simulink model "motion_3D_1_2_w12_5"  (R2025b)
settings: Solver=FixedStepAuto  StartTime=0.0  StopTime=3.5  FixedStep=Ts  RelTol=1e-3
values from neighbouring files (symbols this model uses):
  Ts = 1/1600    (= 0.000625)    [path_control.m]    (also in run_case1.m; run_case1_Cdx.m; run_simulation.m = params.common.Ts; verify_eq12_spectral_PP.m)
libraries: simulink x1, slpidlib x1
settings Model: Creator=user  LastModifiedBy=PME406_01
settings SolverCC: AlgebraicLoopSolver=LineSearch
settings DataIOCC: SaveFormat=Array  ReturnWorkspaceOutputs=off
settings DebuggingCC: UnconnectedInputMsg=warning  UnconnectedOutputMsg=warning  UnconnectedLineMsg=warning  ArithmeticOperatorsInVariantConditions=warning
settings ModelReferenceCC: EnableRefExpFcnMdlSchedulingChecks=on
settings SFSimCC: SimUseLocalCustomCode=off  CustomCodeUndefinedFunction=UseInterfaceOnly
settings RTWCC: RTWUseLocalCustomCode=off  GPUComputeCapability=3.5
settings CodeAppCC: StateflowObjectComments=on

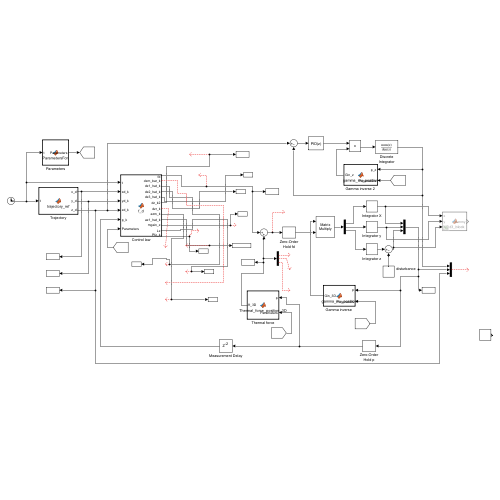
[thumbnail: Simulink's stored preview of the top-level diagram]
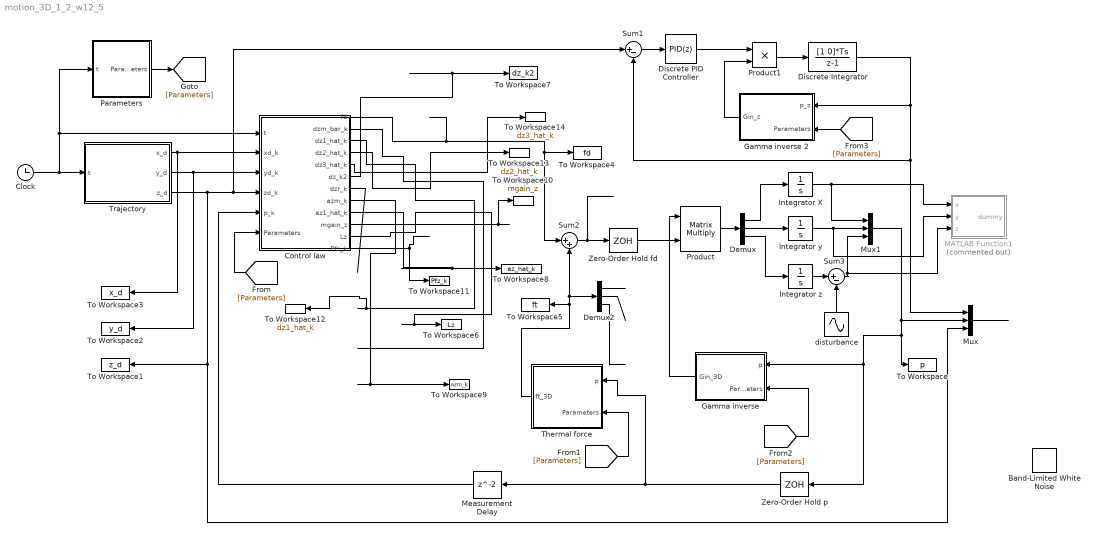
== system motion_3D_1_2_w12_5 ==
  Band-Limited White Noise : simulink/Sources/Band-Limited White Noise  Cov=[0.1]  Ts=0.1  seed=[23341]
  Clock : Clock
  Control law : MATLAB Function  TreatAsAtomicUnit=on
  Demux : Demux  Outputs=3
  Demux2 : Demux  Outputs=3
  Discrete Integrator : DiscreteTransferFcn  Numerator=[1 0]*Ts  Denominator=[1 -1]  SampleTime=Ts
  Discrete PID Controller : slpidlib/PID Controller  Controller=PID  Form=Parallel  TimeDomain=Discrete-time  UseExternalTs=off  SampleTime=Ts  IntegratorMethod=Forward Euler  FilterMethod=Forward Euler  ControllerParametersSource=internal  P=1  I=1  UseKiTs=off  D=0  UseExternalDerivativeSource=off  N=31.4504174128775  UseFilter=on  TunerSelectOption=Transfer Function Based (PID Tuner App)  InitialConditionSource=internal  InitialConditionForIntegrator=0  InitialConditionForFilter=0  DifferentiatorICPrevScaledInput=0  ExternalReset=none  TrackingMode=off  Kt=1  LimitOutput=off  SatLimitsSource=internal  UpperSaturationLimit=inf  LowerSaturationLimit=-inf  LinearizeAsGain=off  AntiWindupMode=none  Kb=1  LimitIntegrator=off  UpperIntegratorSaturationLimit=inf  LowerIntegratorSaturationLimit=-inf  POutMin=[]  POutMax=[]  IOutMin=[]  IOutMax=[]  DOutMin=[]  DOutMax=[]  NOutMin=[]  NOutMax=[]  SumOutMin=[]  SumOutMax=[]  SaturationOutMin=[]  SaturationOutMax=[]  PParamMin=[]  PParamMax=[]  IParamMin=[]  IParamMax=[]  DParamMin=[]  DParamMax=[]  NParamMin=[]  NParamMax=[]  KbParamMin=[]  KbParamMax=[]  KtParamMin=[]  KtParamMax=[]  KbOutMin=[]  KbOutMax=[]  KtOutMin=[]  KtOutMax=[]  IntegratorOutMin=[]  IntegratorOutMax=[]  FilterOutMin=[]  FilterOutMax=[]  SumI1OutMin=[]  SumI1OutMax=[]  SumI2OutMin=[]  SumI2OutMax=[]  SumI3OutMin=[]  SumI3OutMax=[]  SumI4OutMin=[]  SumI4OutMax=[]  SumDOutMin=[]  SumDOutMax=[]  DifferentiatorOutMin=[]  DifferentiatorOutMax=[]  FilterDiffOutCoefMin=[]  FilterDiffOutCoefMax=[]  ReciprocalOutMin=[]  ReciprocalOutMax=[]  SumDenOutMin=[]  SumDenOutMax=[]  SumNumOutMin=[]  SumNumOutMax=[]  DivideOutMin=[]  DivideOutMax=[]  UdiffTsProdOutMin=[]  UdiffTsProdOutMax=[]  NTsProdOutMin=[]  NTsProdOutMax=[]  UintegralTsProdOutMin=[]  UintegralTsProdOutMax=[]  UngainTsProdOutMin=[]  UngainTsProdOutMax=[]  ClampingZeroOutDataTypeStr=Inherit: Inherit via back propagation  ClampingZeroOutMin=[]  ClampingZeroOutMax=[]  FilterDenConstantOutDataTypeStr=Inherit: Inherit via back propagation  FilterDenConstantOutMin=[]  FilterDenConstantOutMax=[]  PCopyOutDataTypeStr=Inherit: Inherit via back propagation  PCopyOutMin=[]  PCopyOutMax=[]  NCopyOutDataTypeStr=Inherit: Inherit via back propagation  NCopyOutMin=[]  NCopyOutMax=[]  IntegratorContinuousStateAttributes=''  IntegratorStateMustResolveToSignalObject=off  IntegratorRTWStateStorageClass=Auto  FilterContinuousStateAttributes=''  FilterStateMustResolveToSignalObject=off  FilterRTWStateStorageClass=Auto  ParallelPVariant=InternalParameters  IdealPVariant=Disabled  IVariant=InternalParameters  DVariant=InternalParameters  IntegratorVariant=Discrete  SatVariant=Disabled  AWVariant=Passthrough  PCopyVariant=Disabled  TRVariant=Disabled  FdbkBlocksVariant=Forward  IdealPFdbkVariant=Disabled  SatFdbkVariant=Disabled  DerivativeFilterVariant=ForwardEulerFilter  NVariant=InternalParameters  NCopyVariant=Disabled  FilterICVariant=InternalICsFilter  IntegratorICVariant=InternalICs  ExternalResetVariant=Disabled  TRSumVariant=Passthrough  SumFdbkVariant=Disabled  SumVariant=Sum_PID  TsampFilterVariant=InternalTs  TsampNgainVariant=Passthrough  TsampIntegralVariant=Disabled_SignalSpec  ExternalSaturationOutDataTypeStr=Inherit: Same as second input  DerivativeSourceVariant=ErrorSignal  PreIntVariant=InternalPreInt
  "Gamma inverse " : MATLAB Function  TreatAsAtomicUnit=on
  "Gamma inverse 2 " : MATLAB Function  TreatAsAtomicUnit=on
  Integrator X : Integrator
  Integrator y : Integrator
  Integrator z : Integrator
  MATLAB Function1 : MATLAB Function  Commented=on  TreatAsAtomicUnit=on
  Measurement Delay : Delay  SampleTime=Ts
  Mux : Mux  Inputs=3
  Mux1 : Mux  Inputs=3
  Parameters : MATLAB Function  TreatAsAtomicUnit=on
  Product : Product  Multiplication=Matrix(*)
  Product1 : Product
  Sum1 : Sum  Inputs=|+-
  Sum2 : Sum  Inputs=|++
  Sum3 : Sum  Inputs=|+-
  "Thermal force " : MATLAB Function  TreatAsAtomicUnit=on
  To Workspace : ToWorkspace  VariableName=p  SampleTime=Ts
  To Workspace1 : ToWorkspace  VariableName=z_d  SampleTime=Ts
  To Workspace10 : ToWorkspace  VariableName=mgain_z  SampleTime=Ts
  To Workspace11 : ToWorkspace  VariableName=Pfz_k  SampleTime=Ts
  To Workspace12 : ToWorkspace  VariableName=dz1_hat_k  SampleTime=Ts
  To Workspace13 : ToWorkspace  VariableName=dz2_hat_k  SampleTime=Ts
  To Workspace14 : ToWorkspace  VariableName=dz3_hat_k  SampleTime=Ts
  To Workspace2 : ToWorkspace  VariableName=y_d  SampleTime=Ts
  To Workspace3 : ToWorkspace  VariableName=x_d  SampleTime=Ts
  To Workspace4 : ToWorkspace  VariableName=fd  SampleTime=Ts
  To Workspace5 : ToWorkspace  VariableName=ft  SampleTime=Ts
  To Workspace6 : ToWorkspace  VariableName=Lz  SampleTime=Ts
  To Workspace7 : ToWorkspace  VariableName=dz_k2  SampleTime=Ts
  To Workspace8 : ToWorkspace  VariableName=az_hat_k  SampleTime=Ts
  To Workspace9 : ToWorkspace  VariableName=azm_k  SampleTime=Ts
  Trajectory : MATLAB Function  TreatAsAtomicUnit=on
  Zero-Order Hold fd : ZeroOrderHold  SampleTime=Ts
  Zero-Order Hold p : ZeroOrderHold  SampleTime=Ts
  "disturbance " : Sin  Amplitude=0*10^-6  Frequency=2*pi*10  Phase=pi/2  SampleTime=Ts
  wires:
  Mux/1 -> ?
  Product1/1 -> Discrete Integrator/1
  Integrator z/1 -> Sum3/1
  Sum3/1 -> MATLAB Function1/3(z), Mux1/3
  Sum1/1 -> Discrete PID Controller/1
  Discrete PID Controller/1 -> Product1/1
  Measurement Delay/1 -> Control law/5(p_k)
  Integrator X/1 -> Mux1/1, MATLAB Function1/1(x)
  Mux1/1 -> Zero-Order Hold p/1, "Gamma inverse "/1(p), To Workspace/1, Mux/2
  Control law/1(fd) -> Sum2/1, To Workspace4/1
  "disturbance "/1 -> Sum3/2
  Integrator y/1 -> MATLAB Function1/2(y), Mux1/2
  Clock/1 -> Parameters/1(t), Control law/1(t), Trajectory/1(t)
  Trajectory/2(y_d) -> To Workspace2/1, Control law/3(yd_k)
  Trajectory/3(z_d) -> Mux/3, To Workspace1/1, Control law/4(zd_k), Sum1/1
  Discrete Integrator/1 -> Mux/1, Sum1/2, "Gamma inverse 2 "/1(p_z)
  Product/1 -> Demux/1
  Trajectory/1(x_d) -> To Workspace3/1, Control law/2(xd_k)
  Demux/1 -> Integrator X/1
  Demux/2 -> Integrator y/1
  Demux/3 -> Integrator z/1
  Zero-Order Hold fd/1 -> Product/2
  Zero-Order Hold p/1 -> "Thermal force "/1(p), Measurement Delay/1
  Sum2/1 -> Zero-Order Hold fd/1
  Demux2/1 -> ?
  Demux2/2 -> ?
  Demux2/3 -> ?
  Control law/6(dz_k2) -> To Workspace7/1
  Control law/2(dzm_bar_k) -> ?
  Control law/7(dzr_k) -> ?
  Control law/3(dz1_hat_k) -> To Workspace12/1
  Control law/8(azm_k) -> To Workspace9/1
  Control law/9(az1_hat_k) -> To Workspace8/1
  Control law/11(Lz) -> To Workspace6/1
  Control law/10(mgain_z) -> To Workspace10/1
  Control law/12(Pfz_k) -> To Workspace11/1
  Control law/4(dz2_hat_k) -> To Workspace13/1
  Control law/5(dz3_hat_k) -> To Workspace14/1
  "Thermal force "/1(ft_3D) -> To Workspace5/1, Demux2/1, Sum2/2
  Parameters/1(Parameters) -> [Parameters]
  [Parameters] -> Control law/6(Parameters)
  [Parameters] -> "Thermal force "/2(Parameters)
  "Gamma inverse "/1(Gin_3D) -> Product/1
  [Parameters] -> "Gamma inverse "/2(Parameters)
  "Gamma inverse 2 "/1(Gin_z) -> Product1/2
  [Parameters] -> "Gamma inverse 2 "/2(Parameters)

== matlab function motion_3D_1_2_w12_5/MATLAB Function1 ==
  data: x input; dummy output; y input; z input
function dummy = plot3_block(x, y, z)
% 用於模擬時即時顯示 3D 點 / 轨跡

% 告訴 codegen：這些函式只在模擬時呼叫
%coder.extrinsic('plot3','figure','hold','grid','xlabel','ylabel','zlabel',...
%                'get','set','drawnow');
coder.extrinsic('plot3','figure','hold','grid','xlabel','ylabel','zlabel',...
                'get','set','drawnow','axis','xlim','ylim','zlim','view','rotate3d');
persistent h
persistent isInit

if isempty(isInit)
    figure; hold on; grid on;
    xlabel('x'); ylabel('y'); zlabel('z');
    axis equal;                   % 三個方向比例一樣
    xlim([-1 1]*4*10^1);                 % 自己設定範圍（依你的資料）
    ylim([-1 1]*4*10^1);
    zlim([-1 1]*4*10^1);
    view(3);                      % 確認使用 3D 視角
    rotate3d on;
    
    % 先畫第一個點，取得圖形 handle
    h = plot3(x, y, z, '.-');
    isInit = true;
else
    % 讀取舊資料，把新的點接到後面
    X = get(h, 'XData');  Y = get(h, 'YData');  Z = get(h, 'ZData');
    X = [X x];  Y = [Y y];  Z = [Z z];
    set(h, 'XData', X, 'YData', Y, 'ZData', Z);
end

drawnow;          % 更新圖形
dummy = 0;        % 給一個不重要的輸出
end

== matlab function motion_3D_1_2_w12_5/Control law ==
  settings: updateMethod=DISCRETE  sampleTime=Ts
  data: t input; xd_k input; yd_k input; zd_k input; fd output size=[3 1]; p_k input size=[3 1]; dzm_bar_k output; dz1_hat_k output; dz2_hat_k output; dz3_hat_k output; dz_k2 output; dzr_k output; azm_k output; az1_hat_k output; mgain_z output; Lz output; Pfz_k output; Parameters input
function [fd, dzm_bar_k, dz1_hat_k, dz2_hat_k, dz3_hat_k, dz_k2 , dzr_k , azm_k , az1_hat_k , mgain_z , Lz , Pfz_k] = f_d(t, xd_k,yd_k,zd_k, p_k, Parameters)

% xd_k : x_d[k]
% xd_k1  : x_d[k-1]
% x_k   : x[k]
% fd    : f_d[k]
% ====================================================================
% PERSISTENT STATE VARIABLES
% ====================================================================
persistent xd_k1                 % x_d[k-1],         - Input history
persistent xd_k2
persistent yd_k1
persistent yd_k2
persistent zd_k1
persistent zd_k2
persistent px_k
persistent py_k
persistent pz_k
persistent fd_X
persistent fd_Y
persistent fd_Z

persistent        dx1_hat_k1
persistent        dx2_hat_k1 
persistent        dx3_hat_k1 
persistent        dz1_hat_k1
persistent        dz2_hat_k1 
persistent        dz3_hat_k1 
persistent        xD_hat_k1 
persistent        dxD_hat_k1
persistent        zD1_hat_k1 
persistent        zD2_hat_k1
persistent        ax_hat_k1 
persistent        ax_hat_k2
persistent        az1_hat_k1 
persistent        az1_hat_k2
persistent        dax_hat_k1 
persistent        az2_hat_k1 
persistent        Pfx_k1
persistent        Pfz_k1
persistent        fd_X_k1 
persistent        fd_X_k2
persistent        fd_Z_k1 
persistent        fd_Z_k2

persistent      dxm_bar_k1
persistent      dxr_bar_k1
persistent     dxr2_bar_k1
persistent      dzm_bar_k1
persistent      dzr_bar_k1
persistent     dzr2_bar_k1

persistent      px_k1
persistent      pz_k1
persistent      PPx_k1
persistent      PPz_k1
%persistent      dx_k1
%persistent      dx_k2
persistent      dx_k3
%persistent      dy_k1
%persistent      dy_k2
persistent      dy_k3
%persistent      dz_k1
%persistent      dz_k2
persistent      dz_k3
persistent      px_bar_k1
persistent      pz_bar_k1
persistent      dxrr_bar_k1
persistent      dzrr_bar_k1
persistent      dxm_k1
persistent      dzm_k1
persistent      azm_k1
% ====================================================================
% INITIALIZATION
% ====================================================================
    if isempty(xd_k1)
        xd_k1 = 0;     % 初始化（第一次執行時）
        xd_k2 = 0;
        yd_k1 = 0;
        yd_k2 = 0;
%        yd_k1 = 6.5;   %um  *10^-6;
        zd_k1 = 0;
        zd_k2 = 0;
        px_k = 0;
        py_k = 0;
        pz_k = 0;
        fd_X = 0;
        fd_Y = 0;
        fd_Z = 0;
        
         xD_hat_k1 = 0;
         
        dx1_hat_k1 = 0; 
        dx2_hat_k1 = 0;
        dx3_hat_k1 = 0;
        dz1_hat_k1 = 0; 
        dz2_hat_k1 = 0;
        dz3_hat_k1 = 0;
        
        xD_hat_k1 = 0;
        dxD_hat_k1 = 0;
        zD1_hat_k1 = 0;
        zD2_hat_k1 = 0;
        
        ax_hat_k1 = 0.012;   %( um/(pN sec))   %ax_normal = 0.0147*10^6; % ( m/(N sec))
        ax_hat_k2 = 0;
        az1_hat_k1 = 0.012/(1+Parameters.beta); % beta=0.5 %( um/(pN sec))        %az_normal = 0.0147*10^6; % ( m/(N sec))
        az_hat_k2 = 0;
        
        dax_hat_k1 = 0;
        az2_hat_k1 = 0;
        
        Pfx_k1 = (0.0147)*4*(1.3806503*10^-23)*(273.15 + 37)*diag([1 1 1 1 1 1 1])*1/4*10^-2;
        
        dz_variance = (2.3*10^-3)^2;    %(um)^2
        Pfz_11 = dz_variance; Pfz_22 = dz_variance;Pfz_33 = dz_variance;
        Pfz_44 = dz_variance;Pfz_55 = dz_variance;
        az_variance = (10^-1*az1_hat_k1)^2;
        Pfz_66 = az_variance; Pfz_77 = az_variance;
       % Pfz_k1 = diag([Pfz_11 Pfz_22 Pfz_33 Pfz_44 Pfz_55 Pfz_66 Pfz_77]);
        
       % simulation by experienced data
        Pfz_11 = Parameters.Pfz_11;
        Pfz_22 = Parameters.Pfz_22;
        Pfz_33 = Parameters.Pfz_33;
        Pfz_44 = Parameters.Pfz_44;
        Pfz_55 = Parameters.Pfz_55;
        Pfz_66 = Parameters.Pfz_66;
        Pfz_77 = Parameters.Pfz_77;
        Pfz_k1 = diag([Pfz_11 Pfz_22 Pfz_33 Pfz_44 Pfz_55 Pfz_66 Pfz_77]);
        
        dxm_bar_k1 = 0;
        dzm_bar_k1 = 0;
        dxr_bar_k1 = 0;
        dzr_bar_k1 = 0;
        dxrr_bar_k1 = 0;
        dzrr_bar_k1 = 0;
        
        dxr2_bar_k1 = 0.9*10^-15;
        
        dzr2_bar_k1 = (0.012*10^6)/Parameters.Am_scaling*4*Parameters.kb*Parameters.T*(2+1/(1-Parameters.lamdaC^2))*(10^6)^2; % (um)^2  ;  azm_n/azm_meas_factor* 4*kb*T * ( 2 + 1/(1 - lamdaC^2) );
        
        fd_X_k1 = 0;    %1*10^-12*10^6;
        fd_X_k2 = 0;
        fd_Z_k1 = 0;    %1*10^-12*10^6;
        fd_Z_k2 = 0;        
        
        px_k1 = 0;
        pz_k1 = 0;
        PPx_k1 = 4*(1.3806503*10^-23)*(273.15 + 37)*0.0147*10^38;        % 4*T*kB*t/g*10^38; da-min 
        PPz_k1 = 4*(1.3806503*10^-23)*(273.15 + 37)*0.0147*10^38;        % 4*T*kB*t/g*10^38;  da-min
%       dx_k1 = 0;     
%       dx_k2 = 0;
        dx_k3 = 0;
 %       dy_k1 = 0;     
 %       dy_k2 = 0;
        dy_k3 = 0;
 %       dz_k1 = 0;     
 %       dz_k2 = 0;
        dz_k3 = 0;        
        px_bar_k1 = 0;
        pz_bar_k1 = 0;
        dxm_k1 =  0;
        dzm_k1 =  0;
        
       azm_k1 = 0.012/Parameters.Am_scaling;  % ( um/(pN sec))   ;az_normal = 0.0147*10^6; %azm_meas_factor=2.5
    end
    
        Ts = Parameters.Ts;
        lamdaC = Parameters.lamdaC;
        gammaN = Parameters.gammaN;

        %parameters
        kb = Parameters.kb;
        T = Parameters.T;
        ax_normal = Parameters.ax_normal;
        az_normal = Parameters.az_normal;

        px_k = p_k(1);
        py_k = p_k(2);
        pz_k = p_k(3);

    % 1) Two angles and one distance defined the orientation and position of the inclined plane
    %theta = pi/2;
    %phi = 0;
    %pz = -15 *10^-6;
    theta = Parameters.theta;
    phi = Parameters.phi;
    pz = Parameters.pz;  

    % 2_1) Plane normal
    w_hat = [cos(theta)*sin(phi);
             sin(theta)*sin(phi);
             cos(phi)];
    % 2_2) Plane x-y unit vector
    u_hat = [-cos(theta)*cos(phi);
             -sin(theta)*cos(phi);
             sin(phi)];
     v_hat = [sin(theta);
             -cos(theta);
             0];
        
    % 3) Outer-product matrix
    W = w_hat * w_hat.';

    % 4-5) Distance and normalized distance
    %R = 2.25 * 10^-6;
    R = Parameters.R;
    h = dot(p_k, w_hat.') - pz;
    hbar = h / R;

    % 6) Correction functions
    invh = 1./hbar;
    invh2 = invh.^2; invh3 = invh.^3; invh4 = invh.^4; invh5 = invh.^5;
    % c_parallel(hbar)
    denom_par = ( 1 ...
                  - (9/16) * invh ...
                  + (1/8)  * invh3 ...
                  - (45/256)* invh4 ...
                  - (1/16) * invh5 );
    c_par = 1 ./ denom_par;

    % c_perp(hbar)
    invh11 = invh.^11; invh12 = invh.^12;
    denom_perp = ( 1 ...
                   - (9/8)   * invh ...
                   + (1/2)   * invh3 ...
                   - (57/100)* invh4 ...
                   + (1/5)   * invh5 ...
                   + (7/200) * invh11 ...
                   - (1/25)  * invh12 );
    c_perp = 1 ./ denom_perp;
    % Final vector for thermal force

		C = c_par*(u_hat+v_hat)+ c_perp*w_hat;
		
    % Calculate variance for each direction
    % Variance = (4 * k_B * T * gamma_N / Ts) * C.^1
    variance_coeff = 4 * kb * T * (gammaN*10^-6) / Ts;							% unit N^2 (using standard MKS unit)
    Variance = variance_coeff * abs((C.^1));

    % Generate random thermal force
    % F_th ~ N(0, Variance) => F_th = sqrt(Variance) .* randn(3,1)
    ft_3D = sqrt(Variance) .* randn(3, 1)*10^12;											% unit : pN
    
    gamma_x = gammaN * c_par;
    gamma_y = gammaN * c_par;
    gamma_z = gammaN * c_perp;
    
    mgain_x = Ts/gamma_x;       %( um/(pN sec))
    mgain_y = Ts/gamma_y;       %( um/(pN sec))
    mgain_z = Ts/gamma_z;       %( um/(pN sec))

    
        % Generate random thermal motion (noise)
   variance_dxt =  4 * kb * T * mgain_x*10^6;    % m^2
   variance_dyt =  4 * kb * T * mgain_y*10^6;    % m^2  
   variance_dzt =  4 * kb * T * mgain_z*10^6;     % m^2
   
       % Measured data with random thermal motion (noise)
 %   px_k = px_k + sqrt(variance_dxt) .* randn(1, 1)*10^6;			% unit : um
 %   py_k = py_k + sqrt(variance_dyt) .* randn(1, 1)*10^6;			% unit : um
 %   pz_k = pz_k + sqrt(variance_dzt) .* randn(1, 1)*10^6;			% unit : um

    % Generate random measurement noise
    Measurement_Variance_x_y = (0.7*10^-9)^2;               % unit : m^2
    Measurement_Variance_z = (2.3*10^-9)^2;                 % unit : m^2
    
    % Measured data with measurement noise
    px_k = px_k + sqrt(Measurement_Variance_x_y) .* randn(1, 1)*10^6;			% unit :um
    py_k = py_k + sqrt(Measurement_Variance_x_y) .* randn(1, 1)*10^6;			% unit : um
    pz_k = pz_k + sqrt(Measurement_Variance_z) .* randn(1, 1)*10^6;				% unit :um

    
    %------- Control law 1: without estimator  -----------
if false
% control effort fd  with known wall surface ::
%fd_X = (gamma_x/Ts) * ( xd_k - lamdaC*xd_k1 - (1 - lamdaC)*px_k );
%fd_Y = (gamma_y/Ts) * ( yd_k - lamdaC*yd_k1 - (1 - lamdaC)*py_k );
%fd_Z = (gamma_z/Ts) * ( zd_k - lamdaC*zd_k1 - (1 - lamdaC)*pz_k );

% control effort fd with unknown wall surface :
fd_X = (gammaN/Ts) * ( xd_k - lamdaC*xd_k1 - (1 - lamdaC)*px_k );   % unit : pN
fd_Y = (gammaN/Ts) * ( yd_k - lamdaC*yd_k1 - (1 - lamdaC)*py_k );   % unit : pN
fd_Z = (gammaN/Ts) * ( zd_k - lamdaC*zd_k1 - (1 - lamdaC)*pz_k );   % unit : pN
fd = [fd_X;fd_Y;fd_Z];
end

    %------- Control law 2: with estimator  -----------
if true
     %parameters
        % kb = 1.3806503*10^-23;              % Boltsmann's constant
		% T = 273.15 + 37;						% Human's temperature
        
    % eqn(13)
    %Real-time variance estimation for Eq.(10) using IIR.
 
        Avar = Parameters.Avar;
        Avar2 = Parameters.Avar2;
        Avar22 = Parameters.Avar22;
        Avar3 = Parameters.Avar3;
        
        dx_k2 = xd_k2 - px_k;         % x tracking error  2-step delayed measurement (paper)
        dy_k2 = yd_k2 - py_k;         % y tracking error  2-step delayed measurement (paper)
        dz_k2 = zd_k2 - pz_k;         % z tracking error  2-step delayed measurement (paper)

        % 2-step delayed measurement (paper)
            dxm_k = dx_k2;     %% unit :um 
            dzm_k = dz_k2;     %% unit :um 
        
    % ----- (9) deterministic component of measured tracking error x-----
    dxm_bar_k = Avar*dxm_k1 + (1-Avar)*dxm_bar_k1;
    % random component: dxr[k] = dxm[k] - dxm_bar[k]
    dxr_k = dxm_k - dxm_bar_k;
    % ----- IIR mean of dxr:  \bar{dxr}[k] -----
    dxr_bar_k = Avar2*dxr_k + (1-Avar2)*dxr_bar_k1;
    dxrr_k = dxr_k - dxr_bar_k;
    %dxrr_bar_k = Avar22*dxrr_k + (1-Avar22)*dxrr_bar_k1;
    dxrr_bar_k = Avar22*dxr_k + (1-Avar22)*dxrr_bar_k1;     %original
    % ----- IIR mean square of dxr:  \overline{dxr^2}[k] -----
    %dxr2_bar_k = Avar3*dxrr_k^2 + (1-Avar3)*dxr2_bar_k1;
    dxr2_bar_k = Avar3*dxr_k^2 + (1-Avar3)*dxr2_bar_k1;     %original
    % ----- (10) variance: sigma^2 = mean_square - mean^2 -----
     sigma2_dxr = dxr2_bar_k - dxrr_bar_k^2;
    % numerical guard (variance should be >=0)
    if sigma2_dxr < 0
        sigma2_dxr = 0;
    end
    % ----- (9) deterministic component of measured tracking error z-----
     %dzm_bar_k = Avar*dzm_k1 + (1-Avar)*dzm_bar_k1;
    dzm_bar_k = Avar*dzm_k + (1-Avar)*dzm_bar_k1;  % bug fixed 20260225
  
    % random component: dzr[k] = dzm[k] - dzm_bar[k]
     %dzr_k = dzm_k - dzm_bar_k;
     dzr_k = dzm_k1 - dzm_bar_k;    % bugfix 0226
     
%CLAMP  將 dzr_k 限制在 [lo, hi]
    dzr_k = min(max(dzr_k, -6*10^-2), 6*10^-2);     %unit : um
     
    % ----- IIR mean of dzr:  \bar{dzr}[k] -----
    dzr_bar_k = Avar2*dzr_k + (1-Avar2)*dzr_bar_k1;
    dzrr_k = dzr_k - dzr_bar_k;
%    dzrr_k = dz_k - dzr_bar_k;

%CLAMP  將 dzrr_k 限制在 [lo, hi]
   % dzrr_k = min(max(dzrr_k, -5*10^-2), 5*10^-2);      %unit : um
    
    %dzrr_bar_k = Avar22*dzrr_k + (1-Avar22)*dzrr_bar_k1;
    dzrr_bar_k = Avar22*dzr_k + (1-Avar22)*dzrr_bar_k1;    %original 

    % ----- IIR mean square of dzr:  \overline{dzr^2}[k] -----
    %dzr2_bar_k = Avar3*dzrr_k^2 + (1-Avar3)*dzr2_bar_k1;
    dzr2_bar_k = Avar3*dzr_k^2 + (1-Avar3)*dzr2_bar_k1;      %original 
    % ----- (10) variance: sigma^2 = mean_square - mean^2 -----
    sigma2_dzr = dzr2_bar_k - dzrr_bar_k^2;
    % numerical guard (variance should be >=0)
    if sigma2_dzr < 0
        sigma2_dzr = 0;
    end    
  
    sigma2_nx = (0.7*10^-3)^2; %unit : um^2 ; variance of measurrement noise in x direction
    sigma2_nz = (2.3*10^-3)^2; %unit : um^2 ; variance of measurrement noise in z direction
   
    den = 4*kb*T * ( 2 + 1/(1 - lamdaC^2) );  %unit : N m
    
    num_x = sigma2_dxr - ( 2/(1 + lamdaC) ) * sigma2_nx; %unit : um^2
    num_z = sigma2_dzr - ( 2/(1 + lamdaC) ) * sigma2_nz; %unit : um^2

    if num_x < 0
        num_x = 0;
    end

    if num_z < 0
        num_z = 0;
    end
    
    %axm_k_dyna = num_x ./ den;   % use ./ to support vector inputs
    %azm_k_dyna = num_z ./ den;   % use ./ to support vector inputs
    axm_k_dyna = (num_x*10^-12) ./ den*(10^6/10^12);   % use ./ to support vector inputs   unit :( um/(pN sec))
    azm_k_dyna = (num_z*10^-12) ./ den*(10^6/10^12);   % use ./ to support vector inputs   unit :( um/(pN sec))
 
if false
%    if t > 0.1
%       axm_k = 2.5*axm_k_dyna;  %scaling
%       azm_k = 2.5*azm_k_dyna;  %scaling
%     else
%        axm_k =ax_normal; % ( m/(N sec))
%        azm_k =az_normal; % ( m/(N sec))
%    end  
end

    axm_k = 2.5*axm_k_dyna;  %scaling
    azm_k = Parameters.Am_scaling*azm_k_dyna;  %scaling
    
% motion gain reasonable range: 0~0.0147
     %azm_k = min(max(azm_k,0),1.5*0.0147);    

%-----estimator for x -------
    %lamdaF = 1.0; %0.999; % 把 P 放大 1/lamdaF 讓濾波器更願意跟著量測的 azm
    lamdaF = Parameters.lamdaF;
    
    e_x1_k = dxm_bar_k - dx1_hat_k1;  % refer to 2025 paper
    e_ax_k = axm_k - ax_hat_k1;
    esti_error = [e_x1_k e_ax_k]';
    H = [1 0 0 0 0 0 0 ; 0 0 0 0 0 1 0];    % eqn(13) Output matrix

    r11 = (0.7*10^-3)^2*Avar; % unit : um^2
    r22 = (10^-3*ax_hat_k1)^2; % unit : ( um/(pN sec))^2
    
    RR = diag([r11 r22]); % Measurement noise covariance
    q11 = 0; 
    q22 = 0; 
    q33 = ax_hat_k1*4*kb*T*10^6*10^12;  % unit : um^2
    q44 =0; 
    q55 = 0; 
tau_az = 100.0;                 % 想要 0.1s 跟隨
K = 1 - exp(-Ts/tau_az);      % 約 0.00623
betaQ = K^2;                   % 約 3.9e-5

q66 = betaQ * r22;             % 讓 az_hat 不會“學到太自信”→ L62 不會掉到 0
q77 = 10 * betaQ * r22;        % (可選) 讓 daz_hat 也能跟著變；太吵就把 10 改成 1~5
    
    Q = diag([q11 q22 q33 q44 q55 q66 q77]); % Measurement noise covariance
    Fe = [   0  1  0  0  0     0             0;
             0  0  1  0  0     0             0;
             0  0  1 -1  0  -fd_X_k1         0;
             0  0  0  1  1     0             0;
             0  0  0  0  1     0             0;
             0  0  0  0  0     1             1;
             0  0  0  0  0     0             1 ];  
    
 %  recursive step1
    S = H*Pfx_k1*H.' + RR;          % innovation covariance (m x m)
% regularize + force symmetry
epsS = 1e-20;
S = 0.5*(S + S.') + epsS*eye(size(S));
    
    % Recommended (numerically stable): avoid explicit inv()
    Lx = (Pfx_k1*H.') / S;          % (n x m), MATLAB solves X = A/B as X = A*inv(B)
 %  recursive step2   
    n = size(Pfx_k1,1);
    I = eye(n);
    Px = (I - Lx*H) * Pfx_k1;
        % Optional (recommended): enforce symmetry to reduce numerical drift
    Px = 0.5*(Px + Px.');
  %  recursive step3   
    Pfx_k = Fe * Px * Fe.' + Q;
        % Optional (recommended): enforce symmetry to reduce numerical drift
    Pfx_k = 0.5*(Pfx_k + Pfx_k.');
    
        % innovation injection term: L[k] * e[k]
    inj = Lx * esti_error;   % 7x1

    dx1_hat_k = dx2_hat_k1 + inj(1);
    dx2_hat_k = dx3_hat_k1 + inj(2);
    dx3_hat_k = lamdaC * dx3_hat_k1 + inj(3);

    xD_hat_k  = xD_hat_k1  + dxD_hat_k1 + inj(4);
    dxD_hat_k = dxD_hat_k1 + inj(5);

    ax_hat_k   = ax_hat_k1   + dax_hat_k1  + inj(6);
    dax_hat_k  = dax_hat_k1  + inj(7);

%-----estimator for z -------
    %e_z1_k = dzm_bar_k1 - dz1_hat_k1;  % refer to 2025 paper
    e_z1_k = dz_k2 - dz1_hat_k1;  % testing0215

    e_az_k = azm_k1 - az1_hat_k1;
    %e_az_k = 0; %testing0215
    esti_error = [e_z1_k e_az_k]';
    H = [1 0 0 0 0 0 0 ; 0 0 0 0 0 1 0];    % eqn(13) Output matrix

    %r11 = az1_hat_k1*4*kb*T*10^0; %-3; %(2.3*10^-9)^2*10^5;
    %r22 =(10^-1*az1_hat_k1)^2;
    r11 = (az1_hat_k1*10^6)*4*kb*T*(10^12)*Parameters.rz11_scaling;  % unit : um^2; 
    r22 =(Parameters.rz22_scaling*az1_hat_k1)^2;            % unit : ( um/(pN sec))^2
    RR = diag([r11 r22]); % Measurement noise covariance
    
    %q11 = 0; %az1_hat_k1*4*kb*T*10^5; 
    %q22 = 0; %az1_hat_k1*4*kb*T*10^5; 
    %q33 = az1_hat_k1*4*kb*T*10^5;
    %q44 = az1_hat_k1*4*kb*T*10^2; %3; %1;
    %q55 = az1_hat_k1*4*kb*T*10^2; %3; %1;

    q11 = (az1_hat_k1*10^6)*4*kb*T*(10^12)*Parameters.qz11_scaling;  % unit : um^2;
    q22 = (az1_hat_k1*10^6)*4*kb*T*(10^12)*Parameters.qz22_scaling;  % unit : um^2;;
    q33 = (az1_hat_k1*10^6)*4*kb*T*(10^12)*Parameters.qz33_scaling;  % unit : um^2;;
    q44 = (az1_hat_k1*10^6)*4*kb*T*(10^12)*Parameters.qz44_scaling;  % unit : um^2;;
    q55 = (az1_hat_k1*10^6)*4*kb*T*(10^12)*Parameters.qz55_scaling;  % unit : um^2;;

    q66 = Parameters.qz66_scaling * r22;
    q77 = Parameters.qz77_scaling * r22;

    %tau_az = 0.15;  %0.1;                 % 想要 0.1s 跟隨
    %K = 1 - exp(-Ts/tau_az);      % 約 0.00623
    %betaQ = K^2;                   % 約 3.9 e-5
    %q66 = betaQ * r22;             % 讓 az_hat 不會“學到太自信”→ L62 不會掉到 0
    %q77 = betaQ * r22;        % (可選) 讓 daz_hat 也能跟著變；太吵就把 10 改成 1~5

    Q = diag([q11 q22 q33 q44 q55 q66 q77]); % Measurement noise covariance

    %beta = 0.5;
    beta = Parameters.beta;
    Fe = [   0  1  0  0         0          0             0;
             0  0  1  0         0          0             0;
             0  0  1 -1         0      -fd_Z_k1          0;
             0  0  0  1+beta  -beta        0             0;
             0  0  0  1         0          0             0;
             0  0  0  0         0         1+beta       -beta;
             0  0  0  0         0          1             0 ];  
    
 %  recursive step1
    S = H*Pfz_k1*H.' + RR;          % innovation covariance (m x m)
% regularize + force symmetry
epsS = 1e-20;
S = 0.5*(S + S.') + epsS*eye(size(S));
    
    % Recommended (numerically stable): avoid explicit inv()
    Lz = (Pfz_k1*H.') / S;          % (n x m), MATLAB solves X = A/B as X = A*inv(B)
 %  recursive step2   
    n = size(Pfz_k1,1);
    I = eye(n);
    Pz = 1/lamdaF * (I - Lz*H) * Pfz_k1;
        % Optional (recommended): enforce symmetry to reduce numerical drift
    Pz = 0.5*(Pz + Pz.');
  %  recursive step3   
    Pfz_k = Fe * Pz * Fe.' + Q;
        % Optional (recommended): enforce symmetry to reduce numerical drift
    Pfz_k = 0.5*(Pfz_k + Pfz_k.');
    
        % innovation injection term: L[k] * e[k]
    inj = Lz * esti_error;   % 7x1

    dz1_hat_k = dz2_hat_k1 + inj(1);
    dz2_hat_k = dz3_hat_k1 + inj(2);
    dz3_hat_k = lamdaC * dz3_hat_k1 + inj(3);

    zD1_hat_k  = (1+beta)* zD1_hat_k1 - beta*zD2_hat_k1 + inj(4);
    zD2_hat_k = zD1_hat_k1 + inj(5);

    az1_hat_k   = (1+beta)* az1_hat_k1 - beta* az2_hat_k1  + inj(6);
    az2_hat_k  = az1_hat_k1  + inj(7);
    
% control effort fd with unknown wall surface :

%%    fd_X = 1/(ax_hat_k) * ( xd_k - xd_k1 + (1 - lamdaC)*dx3_hat_k - xD_hat_k );       % pN
%%    fd_Y = (gammaN/Ts) * ( yd_k - lamdaC*yd_k1 - (1 - lamdaC)*py_k );                   % pN
     fd_Z = 1/(az1_hat_k) * ( zd_k - zd_k1 + (1 - lamdaC)*dz3_hat_k - zD1_hat_k1 );% unit: pN
 
   % conventional control effort without estimator 
 
      fd_X = (1/mgain_x) * ( xd_k - xd_k1 + (1 - lamdaC)*dx_k3);    % pN    2025
      fd_Y = (1/mgain_y) * ( yd_k - yd_k1 + (1 - lamdaC)*dy_k3);    % pN
%%      fd_Z = (1/mgain_z) * ( zd_k - zd_k1 + (1 - lamdaC)*dz_k3);    % pN

fd = [fd_X;fd_Y;fd_Z];
end

% ====================================================================
% STATE UPDATES
% ====================================================================
    xd_k2 = xd_k1;
    xd_k1 = xd_k;
    yd_k2 = yd_k1;
    yd_k1 = yd_k;
    zd_k2 = zd_k1;
    zd_k1 = zd_k;
    
    dx1_hat_k1 = dx1_hat_k;
    dx2_hat_k1 = dx2_hat_k;
    dx3_hat_k1 = dx3_hat_k;
    dz1_hat_k1 = dz1_hat_k;
    dz2_hat_k1 = dz2_hat_k;
    dz3_hat_k1 = dz3_hat_k;
    xD_hat_k1 = xD_hat_k;
    zD1_hat_k1 = zD1_hat_k;
    dxD_hat_k1 = dxD_hat_k;
    zD2_hat_k1 = zD2_hat_k;
    ax_hat_k2 = ax_hat_k1;
    ax_hat_k1 = ax_hat_k;
    az1_hat_k2 = az1_hat_k1;
    az1_hat_k1 = az1_hat_k;
    dax_hat_k1 = dax_hat_k;
    az2_hat_k1 = az2_hat_k;

    Pfx_k1 = Pfx_k;
    Pfz_k1 = Pfz_k;
   
    dxm_bar_k1 = dxm_bar_k;
    dzm_bar_k1 = dzm_bar_k;
    dxr_bar_k1 = dxr_bar_k;
    dxrr_bar_k1 = dxrr_bar_k;
    dxr2_bar_k1 = dxr2_bar_k;
    dzr_bar_k1 = dzr_bar_k;
    dzrr_bar_k1 = dzrr_bar_k;
    dzr2_bar_k1 = dzr2_bar_k;
    
    fd_X_k2 = fd_X_k1;
    fd_X_k1 = fd_X;
    fd_Z_k2 = fd_Z_k1;
    fd_Z_k1 = fd_Z;
    px_k1 = px_k;
    pz_k1 = pz_k;

    dx_k3 = dx_k2;
%    dx_k2 = dx_k1;
%    dx_k1 = dx_k;
    dy_k3 = dy_k2;
%    dy_k2 = dy_k1;
%    dy_k1 = dy_k;
    dz_k3 = dz_k2;
%    dz_k2 = dz_k1;
%    dz_k1 = dz_k;
%    px_bar_k1 = px_bar_k;
%    pz_bar_k1 = pz_bar_k;
     dxm_k1 = dxm_k;
     dzm_k1 = dzm_k;
     azm_k1 = azm_k; 
     
end

== matlab function motion_3D_1_2_w12_5/Trajectory ==
  settings: updateMethod=DISCRETE  sampleTime=Ts
  data: t input; x_d output; y_d output; z_d output
function [x_d, y_d, z_d] = trajectory_ref(t)
%------- curve 1: Da-ming simu code trajectory ----
if  false
rx = 0;     % um  *10^-6;
ry = 0;     % um  *10^-6;*10^-6;
rz = 6.0;     % um   *10^-6;

theta_x = 2*pi*5*t;   % 5 HZ
theta_y = 2*pi*5*t;   % 5 HZ
theta_z = 2*pi*0.8*t;   % 0.8 HZ

x_d = rx * sin(theta_x);
%y_d = ry * sin(theta+pi/2);
y_d = ry * sin(theta_y);
z_d = -rz + rz * cos(theta_z);

end

%------- curve 1-2: Da-ming fixed trajectory ----
if  true
rx = 0;     % um  *10^-6;
ry = 0;     % um  *10^-6;
rz = 6.0;     % um  *10^-6;
theta_x = 2*pi*5*t;   % 5 HZ
theta_y = 2*pi*5*t;   % 5 HZ

if t < 1.5
%if t < 15
z_d = 0;
elseif t < 2.75
theta_z = 2*pi*0.4*(t-1.5);   % 0.4 HZ
z_d = -rz + rz * cos(theta_z);
else 
z_d = -2*rz;
   
end

x_d = rx * sin(theta_x);
%y_d = ry * sin(theta+pi/2);
y_d = ry * sin(theta_y);
%z_d = -rz + rz * cos(theta_z);

end

%------- curve 2: 8 shape trajectory ----
if  false
rx = 6;     % um  *10^-6;
ry = 6;     % um  *10^-6;
rz = 12.7;     % um  *10^-6;

theta = 2*pi*1*t;   % 1 HZ

x_d = rx * sin(theta);
%y_d = ry * sin(theta+pi/2);
y_d = ry * sin(2*theta);
z_d = rz * sin(theta);

end

if false
%------ curve 3: 螺旋/轉向軌跡 trajectory ------------

%% Parameters
N      = 5;        % number of cycles
Tc     = 0.35;     % seconds per cycle
Tup    = N*Tc;     % 1.75 s
Tdown  = 0.25;     % return time
Ttot   = Tup + Tdown;

Rmax   = 30;     % um  *10^-6;       % um (final radius)
Zmax   = 15;     % um  *10^-6;       % um (final height)

%% Allocate

s1  = t / Tup;  

theta = 2*pi*N*s1;              % total 5 turns
r     = Rmax*s1;

if t <= Tup
theta = 2*pi*N*s1;              % total 5 turns
r     = Rmax*s1;
x_d = r .* cos(theta);
y_d = r .* sin(theta);
z_d = Zmax*s1;
elseif t< Ttot
s2=(t - Tup) / Tdown
x_d = Rmax*(1 - s2);
y_d = 0;
z_d = Zmax*(1 - s2);    
else
x_d = 0;
y_d = 0;
z_d = 0;     
end

end

end

== matlab function motion_3D_1_2_w12_5/Parameters ==
  settings: updateMethod=DISCRETE  sampleTime=Ts
  data: t input; Parameters output Bus: ParametersBus
function Parameters  = ParametersFcn(t)

% --- Controller --------
    Parameters.Ts = 1/1600;
    Parameters.lamdaC = 0.7;
% --- Two angles and one distance defined the orientation and position of the inclined plane --------
    Parameters.theta = pi/2;
    Parameters.phi = 0;
    Parameters.pz = -15;            % unit : um    
% --- Radius of the magnetic particle --------
    Parameters.R = 2.25;            % unit : um  
% --- Thermal force / motion --------
    Parameters.kb = 1.3806503*10^-23;   % unit : N m / T
    Parameters.T = 273.15 + 37;         % unit :  T
    Parameters.ax_normal = 0.0147;  % unit : ( um/(pN sec))
    Parameters.az_normal = 0.0147;  % unit : ( um/(pN sec))
    Parameters.gammaN = 0.0425;     % unit : (( pN sec)/um)
% --- IIR filter for deterministic component of tracking error --------
    Parameters.Avar = 0.45; %0.15;
    Parameters.Avar2 = 0.005; % not used
    Parameters.Avar22 = 0.05; % 0.1;
    Parameters.Avar3 = 0.05;  % 0.1;
    Parameters.Am_scaling = 10; %4.75; %2.5;
% --- w1_w2 estimator --------
    Parameters.beta = 0.5; 
% --- Kalman filter for z --------
    Parameters.lamdaF = 1;  % forgetting factor;  P 放大 1/lamdaF 讓濾波器更願意跟著量測的 azm

    Parameters.Pfz_11 = 0;                  %unit : um^2
    Parameters.Pfz_22 = 0;                  %unit : um^2
    Parameters.Pfz_33 = 1e-4;               %unit : um^2
    Parameters.Pfz_44 = 1e-4;               %unit : um^2
    Parameters.Pfz_55 = 0;                  %unit : um^2
    Parameters.Pfz_66 = 10*(0.0147)^2;      %unit : ( um/(pN sec))^2
    Parameters.Pfz_77 = 0;                  %unit : ( um/(pN sec))^2
    
    Parameters.rz11_scaling = 10^0;         % base:(az1_hat_k1*10^6)*4*kb*T*(10^12)  unit : um^2
    Parameters.rz22_scaling = 10^-1;        % base:(az1_hat_k1)^2                   unit : ( um/(pN sec))^2
    
    Parameters.qz11_scaling = 0;           % base:(az1_hat_k1*10^6)*4*kb*T*(10^12)  unit : um^2
    Parameters.qz22_scaling = 0;           % base:(az1_hat_k1*10^6)*4*kb*T*(10^12)  unit : um^2
    Parameters.qz33_scaling = 10^4;        % base:(az1_hat_k1*10^6)*4*kb*T*(10^12)  unit : um^2
    Parameters.qz44_scaling = 10^2;        % base:(az1_hat_k1*10^6)*4*kb*T*(10^12)  unit : um^2
    Parameters.qz55_scaling = 0;           % base:(az1_hat_k1*10^6)*4*kb*T*(10^12)  unit : um^2
    Parameters.qz66_scaling = 8*10^-5;     % base:r22                               unit : ( um/(pN sec))^2
    Parameters.qz77_scaling = 0;           % base:r22                               unit : ( um/(pN sec))^2
    
end

== matlab function motion_3D_1_2_w12_5/Thermal force  ==
  settings: updateMethod=DISCRETE  sampleTime=Ts
  data: p input size=[3 1]; ft_3D output size=[3 1]; Parameters input
function ft_3D = Thermal_force_position_3D(p, Parameters)
%function ft_3D = Thermal_force_position_3D(p)
    % 1) Two angles and one distance defined the orientation and position of the inclined plane 
    %theta = pi/2;
    %phi = 0;
    %pz = -15*10^-6;  %unit m
    theta = Parameters.theta;
    phi = Parameters.phi;
    pz = Parameters.pz;    %unit um
    
    % 2_1) Plane normal
    w_hat = [cos(theta)*sin(phi);
             sin(theta)*sin(phi);
             cos(phi)];
    % 2_2) Plane x-y unit vector
    u_hat = [-cos(theta)*cos(phi);
             -sin(theta)*cos(phi);
             sin(phi)];
     v_hat = [sin(theta);
             -cos(theta);
             0];

    % 3) Outer-product matrix
    W = w_hat * w_hat.';

    % 4-5) Distance and normalized distance
    %R = 2.25 * 10^-6;
    R = Parameters.R;
    %gammaN = 0.0425;		% pN sec/um
    gammaN = Parameters.gammaN;     % pN sec/um
    
%    p = [0;0;p_z];
    h = dot(p, w_hat.') - pz;
    hbar = h / R;

    % 6) Correction functions
    invh = 1./hbar;
    invh2 = invh.^2; invh3 = invh.^3; invh4 = invh.^4; invh5 = invh.^5;
    % c_parallel(hbar)
    denom_par = ( 1 ...
                  - (9/16) * invh ...
                  + (1/8)  * invh3 ...
                  - (45/256)* invh4 ...
                  - (1/16) * invh5 );
    c_par = 1 ./ denom_par;

    % c_perp(hbar)
    invh11 = invh.^11; invh12 = invh.^12;
    denom_perp = ( 1 ...
                   - (9/8)   * invh ...
                   + (1/2)   * invh3 ...
                   - (57/100)* invh4 ...
                   + (1/5)   * invh5 ...
                   + (7/200) * invh11 ...
                   - (1/25)  * invh12 );
    c_perp = 1 ./ denom_perp;

    % Final vector

		C = c_par*(u_hat+v_hat)+ c_perp*w_hat;
		%kb = 1.3806503*10^-23;		% Boltsmann's constant
		%T = 273.15+ 37;						% Human's temperature
        kb = Parameters.kb;
        T = Parameters.T;
        
		%Ts = 1/1600;							% sampling time
		 Ts = Parameters.Ts;							% sampling time
		
    % Calculate variance for each direction
    % Variance = (4 * k_B * T * gamma_N / Ts) * C.^1
    variance_coeff = 4 * kb * T * (gammaN*10^-6) / Ts;							% unit N^2 (using standard MKS unit)
    Variance = variance_coeff * abs((C.^1));

    % Generate random thermal force
    % F_th ~ N(0, Variance) => F_th = sqrt(Variance) .* randn(3,1)
    ft_3D = sqrt(Variance) .* randn(3, 1)*10^12;											% unit : pN
%     ft_3D = 0 .* randn(3, 1)*10^9;
end

== matlab function motion_3D_1_2_w12_5/Gamma inverse  ==
  settings: updateMethod=DISCRETE  sampleTime=Ts
  data: p input size=[3 1]; Gin_3D output size=[3 3]; Parameters input
function Gin_3D = gamma_inv_position(p, Parameters)

    % 1) Two angles and one distance defined the orientation and position of the inclined plane 
    %theta = pi/2;
    %phi = 0;
    %pz = -15*10^-6;  

    theta = Parameters.theta;
    phi = Parameters.phi;
    pz = Parameters.pz;  

    % 2) Plane normal
    w_hat = [cos(theta)*sin(phi);
             sin(theta)*sin(phi);
             cos(phi)];

    % 3) Outer-product matrix
    W = w_hat * w_hat.';

    % 4-5) Distance and normalized distance
    %R = 2.25 * 10^-6;
    R = Parameters.R;
    %gammaN = 0.0425;
    gammaN = Parameters.gammaN;
%    p = [0;0;p_z];
    h = dot(p, w_hat.') - pz;
    hbar = h / R;

    % 6) Correction functions
    invh = 1./hbar;
    invh2 = invh.^2; invh3 = invh.^3; invh4 = invh.^4; invh5 = invh.^5;
    % c_parallel(hbar)
    denom_par = ( 1 ...
                  - (9/16) * invh ...
                  + (1/8)  * invh3 ...
                  - (45/256)* invh4 ...
                  - (1/16) * invh5 );
    c_par = 1 ./ denom_par;

    % c_perp(hbar)
    invh11 = invh.^11; invh12 = invh.^12;
    denom_perp = ( 1 ...
                   - (9/8)   * invh ...
                   + (1/2)   * invh3 ...
                   - (57/100)* invh4 ...
                   + (1/5)   * invh5 ...
                   + (7/200) * invh11 ...
                   - (1/25)  * invh12 );
    c_perp = 1 ./ denom_perp;

    % Final matrix
    I = eye(3);
    coeff = 1 / (gammaN * c_par);
    alpha = (c_perp - c_par) / c_perp;
    Gin = coeff * ( I - alpha * W );

%		Gin_z = Gin(3,3);
		Gin_3D = Gin;

end

== matlab function motion_3D_1_2_w12_5/Gamma inverse 2  ==
  settings: updateMethod=DISCRETE  sampleTime=Ts
  data: p_z input; Gin_z output; Parameters input
function Gin_z = gamma_inv_position(p_z, Parameters)

    % 1) Two angles and one distance defined the orientation and position of the inclined plane 
    %theta = pi/2;
    %phi = 0;
    %pz = -15*10^-6;  

    theta = Parameters.theta;
    phi = Parameters.phi;
    pz = Parameters.pz;  
    
    % 2) Plane normal
    w_hat = [cos(theta)*sin(phi);
             sin(theta)*sin(phi);
             cos(phi)];

    % 3) Outer-product matrix
    W = w_hat * w_hat.';

    % 4-5) Distance and normalized distance
    %R = 2.25 * 10^-6;
    R = Parameters.R;
    %gammaN = 0.0425;
    gammaN = Parameters.gammaN;
    p = [0;0;p_z];
    h = dot(p, w_hat.') - pz;
    hbar = h / R;

    % 6) Correction functions
    invh = 1./hbar;
    invh2 = invh.^2; invh3 = invh.^3; invh4 = invh.^4; invh5 = invh.^5;
    % c_parallel(hbar)
    denom_par = ( 1 ...
                  - (9/16) * invh ...
                  + (1/8)  * invh3 ...
                  - (45/256)* invh4 ...
                  - (1/16) * invh5 );
    c_par = 1 ./ denom_par;

    % c_perp(hbar)
    invh11 = invh.^11; invh12 = invh.^12;
    denom_perp = ( 1 ...
                   - (9/8)   * invh ...
                   + (1/2)   * invh3 ...
                   - (57/100)* invh4 ...
                   + (1/5)   * invh5 ...
                   + (7/200) * invh11 ...
                   - (1/25)  * invh12 );
    c_perp = 1 ./ denom_perp;

    % Final matrix
    I = eye(3);
    coeff = 1 / (gammaN * c_par);
    alpha = (c_perp - c_par) / c_perp;
    Gin = coeff * ( I - alpha * W );

		Gin_z = Gin(3,3);

end
